simulink model "dof5mani"  (Simulink 7.9)
settings: Solver=ode3  StartTime=0.0  StopTime=inf  FixedStep=0.01  RelTol=1e-3
libraries: simulink x1
settings Model: Creator=Kadir  LastModifiedBy=Kadir

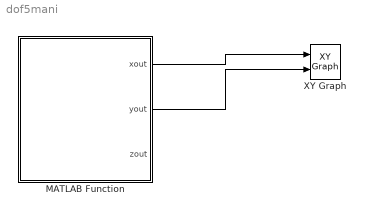
== system dof5mani ==
  MATLAB Function : MATLAB Function  TreatAsAtomicUnit=on
  XY Graph : simulink/Sinks/XY Graph  xmin=-100  xmax=100  ymin=-100  ymax=100  st=-1
  wires:
  MATLAB Function/1(xout) -> XY Graph/1
  MATLAB Function/2(yout) -> XY Graph/2

== matlab function MATLAB Function ==
  data: xout output double; yout output double; zout output double
function [xout,yout,zout] = dof5()
persistent xdes;
if isempty(xdes)
    xdes = 10; % initalize the persistent variable
end
persistent ydes;
if isempty(ydes)
    ydes = 10; % initalize the persistent variable
end
persistent zdes;
if isempty(zdes)
    zdes = 30; % initalize the persistent variable
end
persistent d5;
if isempty(d5)
    d5 = 5; % initalize the persistent variable
end
%application

teta1 = atan2(ydes, xdes) - pi;

if(abs(sin(teta1)) > abs(cos(teta1))) % acinin hangi degeri daha buyukse onunla islem yapalim
       teta2 = atan2((ydes / sin(teta1)), zdes) ;
else
      teta2 = atan2((xdes / cos(teta1)), zdes) ;
end

length = zdes / cos(teta2);
    if(length <= 0);
     %disp('There is an error with decoupled kinematics');
    end;
teta1_deg = teta1 * 180 / pi;
teta2_deg = teta2 * 180 / pi;
PTM = [d5*cos(teta1)*cos(teta2) d5*cos(teta1)*sin(teta2) d5*sin(teta1); d5*sin(teta1)*cos(teta2) d5*sin(teta1)*sin(teta2) -d5*cos(teta1); -d5*sin(teta2) d5*cos(teta2) 0];
%PTM = subs(PTM, [t1 t2 d5], [teta1 teta2 pen_length]);

    if (det(PTM) ~= 0) 
     PTM_inv = PTM^(-1);
    else
     PTM_inv = pinv(PTM);
    end
    
    pen_variable = PTM_inv * [0 d5 0]';
    
    teta5 = asin(pen_variable(3));
    teta4 = atan2(pen_variable(2),pen_variable(1));
    
    teta5_deg = teta5 * 180 / pi;
    teta4_deg = teta4 * 180 / pi;
    
    d2 = 0;d3 = length; t1 =teta1; t2= teta2;

 
Jacob_v = [ -d2*cos(teta1)-d3*sin(teta1)*sin(teta2) d3*cos(teta1)*cos(teta2) cos(teta1)*sin(teta2);d3*cos(teta1)*sin(teta2)-d2*sin(teta1) d3*cos(teta2)*sin(teta1) sin(teta1)*sin(teta2);0 cos(teta1)*(d2*sin(teta1)-d3*cos(teta1)*sin(teta2))-sin(teta1)*(d2*cos(teta1)+d3*sin(teta1)*sin(teta2)) cos(teta2)];

   Jacob_v = subs(Jv, [d2 d3 t1 t2], [0 length teta1 teta2])
    if(det(Jacob_v) ~= 0)
    v = ((Jacob_v)^(-1)) * [0 1 0]'    
    else
    v = (pinv(Jacob_v)) * [0 1 0]'
    end
    teta1  = v(1)*0.001 + teta1
    teta2  = v(2)*0.001 + teta2
    length = v(3)*0.001 + length
    subs(P30, [d1 d2 t1 t2 d3], [0 0 teta1 teta2 length])
   %Jacob_v = subs(Jv, [d2 d3 t1 t2], [0 length teta1 teta2])
    v = Jacob_v * [0 -1 0]'
    xdes = v(1)*0.01 + xdes
    ydes = v(2)*0.01 + ydes
    zdes = v(3)*0.01 + zdes
    
    xout= xdes
    yout= ydes
    zout= zdes;
    
   % plot(xdes,ydes);
    %hold on;

end
